simulink model "modelOfTower"  (R2022a)
settings: Solver=VariableStepAuto  StartTime=0.0  StopTime=50  RelTol=1e-3
libraries: simulink x1
settings Model: Creator=Luc  LastModifiedBy=Luc

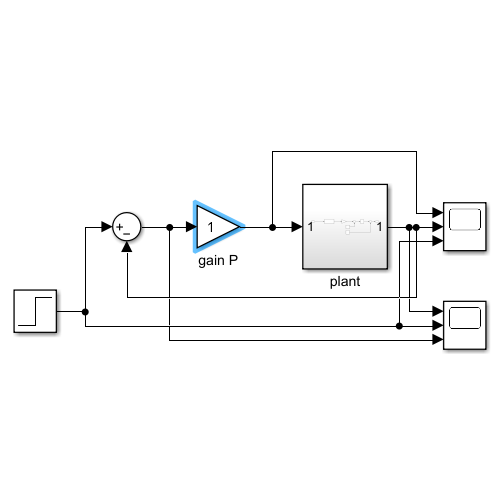
[thumbnail: Simulink's stored preview of the top-level diagram]
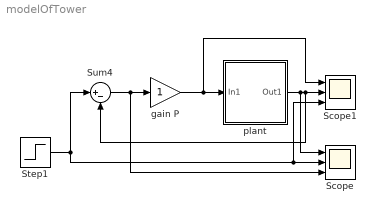
== system modelOfTower ==
  Scope : Scope  NumInputPorts=3
  Scope1 : Scope  NumInputPorts=3
  Step1 : Step  After=5  SampleTime=0
  Sum4 : Sum  Inputs=|+-
  gain P : Gain
  plant : Subsystem
  wires:
  gain P/1 -> Scope1/1, plant/1(In1)
  Sum4/1 -> gain P/1, Scope/3
  plant/1(Out1) -> Sum4/2, Scope1/2, Scope/1
  Step1/1 -> Scope1/3, Scope/2, Sum4/1

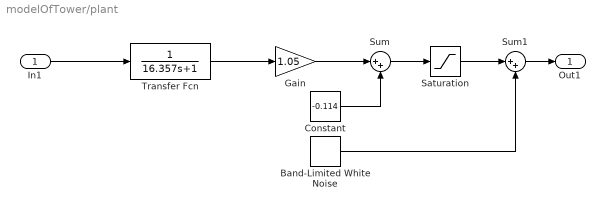
== system modelOfTower/plant ==
  In1 : Inport
  Band-Limited White Noise : simulink/Sources/Band-Limited White Noise  Cov=[0.0001]  Ts=0.01  seed=[23341]
  Constant : Constant  Value=-0.114
  Gain : Gain  Gain=1.05
  Saturation : Saturate  UpperLimit=8.79  LowerLimit=1.206
  Sum : Sum  Inputs=|++
  Sum1 : Sum  Inputs=|++
  Transfer Fcn : TransferFcn  Denominator=[16.357 1]
  Out1 : Outport
  wires:
  Gain/1 -> Sum/1
  Sum1/1 -> Out1/1
  Saturation/1 -> Sum1/1
  Constant/1 -> Sum/2
  Transfer Fcn/1 -> Gain/1
  Band-Limited White Noise/1 -> Sum1/2
  Sum/1 -> Saturation/1
  In1/1 -> Transfer Fcn/1
